simulink library "single_2_bool"  (R2016b)
settings: Solver=VariableStepAuto  StartTime=0.0  StopTime=10.0  RelTol=1e-3
undefined symbols (not defined in the file or in its folder): fsw_params
settings Model: Creator=taylorreynolds  LastModifiedBy=taylorreynolds

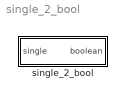
== system single_2_bool ==
  single_2_bool : Subsystem

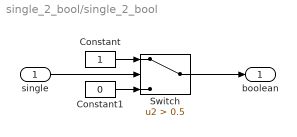
== system single_2_bool/single_2_bool ==
  single : Inport
  Constant : Constant  OutDataTypeStr=boolean  SampleTime=fsw_params.sample_time_s
  Constant1 : Constant  Value=0  OutDataTypeStr=boolean  SampleTime=fsw_params.sample_time_s
  Switch : Switch  Criteria=u2 > Threshold  Threshold=0.5
  boolean : Outport
  wires:
  Constant1/1 -> Switch/3
  single/1 -> Switch/2
  Switch/1 -> boolean/1
  Constant/1 -> Switch/1
